simulink library "MatlabHeatLib"  (Simulink 8.6)
settings: Solver=ode45  StartTime=0.0  StopTime=10.0  RelTol=1e-3
undefined symbols (not defined in the file): ts
libraries: MatlabHeatLib x4, simulink x3
settings Model: Creator=Kai  LastModifiedBy=abp412  ModifiedHistory=Version 2.0 09.05.2011 10:37 Aktuelle Version der MatlabHeatLib

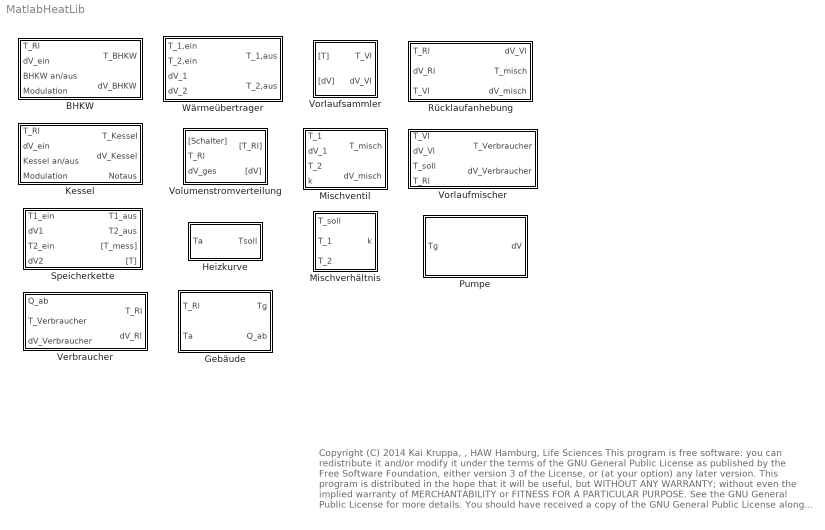
== system MatlabHeatLib ==
  note: Copyright (C) 2014 Kai Kruppa, , HAW Hamburg, Life Sciences
      |
      |     This program is free software: you can redistribute it and/or modify it under the terms of the GNU General Public License
      | as published by the Free Software Foundation, either version 3 of the License, or (at your option) any later version.
      |
      | This program is distributed in the hope that it will be useful, but WITHOUT ANY WARRANTY;
      | without even the implied warranty of MERCHANTABILITY or FITNESS FOR A PARTICULAR PURPOSE.
      | See the GNU General Public License for more details.
      |
      |     You should have received a copy of the GNU General Public License along with this program.  If not, see <http://www.gnu.org/licenses/>.
      |
      | Contact: kai.kruppa@haw-hamburg.de
  BHKW : Subsystem  mask(BHKW){V_BHKW=1.02, P_min=100, P_max=200, k_BHKW=2681, c=4182, rho=1000, BHKWInit=273+70, T_Umgebung=273+30}
      mask prompts: V_BHKW "Volumen [m^3]"; P_min "minimale Leistung [kW]"; P_max "maximale Leistung [kW]"; k_BHKW "Verlustleistungskoeffizient [kW/K]"; c "spez. Wärmekapazität [J/(kg*K)]"; rho "Dichte [kg/m^3]"; BHKWInit "Anfangstemperatur [K]"; T_Umgebung "Umgebungstemperatur [K]"
      mask help:
      | Eingänge:
      | - T_Rl, dV_ein:  Volumenstrom dV_ein mit der Temperatur T_Rl
      | - BHKW an/aus: öffnet und schließt das Ventil des BHKW's
      | - Modulation:     variiert die zugeführte Leistung Q_zu,
      |                         das Signal liegt im Intervall [0,1]
      | Augänge:
      | -T_BHKW, dV_BHKW: Wasser fließt mit einem Volumenstrom
      |                                 dV_BHKW und der Temperatur T_BHKW ab
      | Die Berechnung der Ausgangstemperatur erfolgt über die
      | Wärmeleistungsbilanz:
      | dQ_BHKW = dQ_zu - dQ_Verlust + dQ_BHKW,Rl - dQ_BHKW,Vl
      | Die zugeführte Leistung Q_zu wird auf eine minimale und eine
      | maximale Leistung begrenzt. Ist das BHKW ausgeschaltet, fließt
      | kein Volumenstrom durch die Komponente.
      | Entwickelt auf Grundlage der Bachelorarbeit "Vergleich
      | verschiedener Wärmeversorgungssysteme", 2010 von Herrn Kai
      | Kruppa.
      |
      | Copyright (C) 2014 Kai Kruppa, HAW Hamburg, Life Sciences,
      | GNU General Public License
  Gebäude : Subsystem  mask(Gebäude){kg=0, krg=0, kga=0, TgInit=0}
      mask prompts: kg "Wärmekapazität"; krg "Wärmeübvergnagskoeffizient (Heizung -> Gebäude)"; kga "Wärmeübvergnagskoeffizient (Gebäude -> Umgebung)"; TgInit "Anfangswert der Gebäudetemperatur [K]"
      mask help:
      | Eingänge:
      | - T_Rl: Rücklauftemperatur
      | - Ta:  Außentemperatur
      |
      | Ausgänge:
      | - Tg: Gebäudetemperatur
      | - Q_ab: Wärmeleistungsbedarf
      | Das Gebäude wird als 1 Zonen Modell angenommen. Die
      | Berechnung der Gebäudetemperatur erfolgt über die
      | Wärmeleistungsbilanz
      | kg*dTg = krg(T_Rl-Tg)-kga(Tg-Ta).
      | Der Wärmeleistungsbedarf lautet
      | Q_ab = krg(T_Rl-Tg).
      | Entwickelt auf Grundlage von "Tensor Systems: Multilinear
      | Modeling and Applications", 3rd Int. Conference on Simulation
      | and Modeling Methodologies, Technologies and Applications,
      | 2013, Pangalos, G., Eichler, A., Lichtenberg, G.
      |
      | Copyright (C) 2014 Kai Kruppa, HAW Hamburg, Life Sciences,
      | GNU General Public License
  Heizkurve : Subsystem  mask(Heizkurve){Ta1c=20, Ta2c=-12, Ts1c=60, Ts2c=85}
      mask prompts: Ta1c "Ta1 [°C]"; Ta2c "Ta2 [°C]"; Ts1c "Tsoll1 [°C]"; Ts2c "Tsoll2 [°C]"
      mask help:
      | Eingang:
      | -Ta: Aussentemperatur
      | Ausgang:
      | -Tsoll: Vorlaufsolltemperatur
      | Anhand der Außentemperatur wird über eine gesättigte lineare
      | Heizkurve die Vorlaufsolltemperatur bestimmt. Die Heizkurve wird
      | durch zwei Punkte, die als Parameter angegeben werden,
      | bestimmt.
      |          Tsoll
      |            |
      | Tsoll2 _| _______
      |            |               \
      |            |                  \
      |            |                     \
      | Tsoll1 _|                        \________
      |            |
      |            |_______________________Ta
      |                          |           |
      |                        Ta2        Ta1
      | Entwickelt auf Grundlage der Bachelorarbeit "Vergleich
      | verschiedener Wärmeversorgungssysteme", 2010 von Herrn Kai
      | Kruppa.
      |
      | Copyright (C) 2014 Kai Kruppa, HAW Hamburg, Life Sciences,
      | GNU General Public License
      mask init:
      | Ta1=Ta1c+273.15;
      | Ta2=Ta2c+273.15;
      | Ts1=Ts1c+273.15;
      | Ts2=Ts2c+273.15;
  Kessel : Subsystem  mask(Kessel){V_Kessel=2, P_min=200, P_max=15000, k_Kessel=5000, c=4182, rho=1000, notaustemp=273+95, notauszeit=10, KesselInit=273+70, T_Umgebung=273+30}
      mask prompts: V_Kessel "Volumen [m^3]"; P_min "Minimale Leistung [kW]"; P_max "Maximale Leistung [kW]"; k_Kessel "Verlustleistungsfaktor [W/K]"; c "Spez. Wärmekapazität [J/(kg*K)]"; rho "Dichte [kg/m^3]"; notaustemp "Notaustemperatur [K]"; notauszeit "Notauszeit [s]"; KesselInit "Anfangstemperatur [K]"; T_Umgebung "Umgebungstemperatur [K]"
      mask help:
      | Eingänge:
      | - T_Rl, dV_ein:  Volumenstrom dV_ein mit der Temperatur T_Rl
      | - Kessel an/aus: schaltet die zugeführte Leistung Q_zu an oder ab
      | - Modulation:     variiert die zugeführte Leistung Q_zu,
      |                         das Signal liegt im Intervall [0,1]
      | Augänge:
      | -T_Kessel, dV_Kessel: das erhitzte Wasser fließt mit einem
      |                                  Volumenstrom dV_Kessel und der
      |                                  Temperatur T_Kessel wieder ab
      | -Notaus:                     gibt an, ob der Kessel sich im
      |                                  Notausbetrieb befindet
      | Die Berechnung der Ausgangstemperatur erfolgt über die
      | Wärmeleistungsbilanz:
      | dQ_Kessel = dQ_zu - dQ_Verlust + dQ_Kessel,Rl - dQ_Kessel,Vl
      | Die zugeführte Leistung Q_zu wird auf eine minimale und eine
      | maximale Leistung begrenzt.
      | Sonderfälle:
      | Volumenstrom dV_ein beträgt 0: kein Wasser fließt durch den
      | Kessel -> das im Kessel befindliche Wasser heizt sich auf.
      | Notausbetrieb: T_Kessel > Notaustemperatur -> Q_zu = 0 für
      | die Dauer der Notauszeit.
      | Entwickelt auf Grundlage der Bachelorarbeit "Vergleich
      | verschiedener Wärmeversorgungssysteme", 2010 von Herrn Kai
      | Kruppa.
      |
      | Copyright (C) 2014 Kai Kruppa, HAW Hamburg, Life Sciences,
      | GNU General Public License
  Mischventil : Subsystem  mask(Mischventil){}
      mask help:
      | Es handelt sich um ein 3-Wege-Mischventil.
      | Eingänge:
      | -T_1, dV_1: Temperatur und Volumenstrom des ersten Stromes
      | -T_2:           Temperatur des zweiten Volumenstromes
      | -k:               Mischverhältnis
      | Ausgänge:
      | -T_misch, dV_misch: Temperatur und Volumenstrom des Mischprodukts
      | Dem Volumenstrom dV1 kann, abhängig vom Mischverhältnis k, Wasser
      | aus einem zweiten Volumenstrom dV2 beigemischt werden. Das
      | Mischverhältnis ist auf den Volumenstrom dV1 bezogen.
      | k = dV_2/dV_1
      | Für das Mischprodukt ergibt sich:
      | dV_misch = (1 + k)*dV_1,
      | T_misch = (T_1 + k*T_2)/(1+k).
      | Entwickelt auf Grundlage der Bachelorarbeit "Vergleich verschiedener
      | Wärmeversorgungssysteme", 2010 von Herrn Kai Kruppa.
      |
      | Copyright (C) 2014 Kai Kruppa, HAW Hamburg, Life Sciences,
      | GNU General Public License
  Mischverhältnis : Subsystem  mask(Mischverhältnis){}
      mask help:
      | Eingänge:
      | -T_soll: Vorlaufsolltemperatur
      | -T_1:    Temperatur des Volumenstroms 1
      | -T_2:    Temperatur des Volumenstroms 2
      | Ausgang:
      | -k: Mischverhältnis
      | Es wird berechnet, wieviel Wasser durch den Volumenstrom 2 dem
      | Volumenstrom 1 zugeführt werden muss, um eine gewünschte
      | Temperatur des Mischprodukts zu erhalten. Die gewünschte
      | Temperatur wird durch die Solltemperatur vorgegeben.
      | Das Mischverhältinis k berechnet sich aus
      | k = (T_1-T_soll)/(T_soll-T_2).
      | Entwickelt auf Grundlage der Bachelorarbeit "Vergleich verschiedener
      | Wärmeversorgungssysteme", 2010 von Herrn Kai Kruppa.
      |
      | Copyright (C) 2014 Kai Kruppa, HAW Hamburg, Life Sciences,
      | GNU General Public License
  Pumpe : Subsystem  mask(Pumpe){dVm=0, dVa=0, Tg_soll=0, DeltaTg=0}
      mask prompts: dVm "Mittlerer Volumenstrom [m^3/s]"; dVa "Volumenstromamplitude [m^3/s]"; Tg_soll "Soll-Gebäudetemperatur [K]"; DeltaTg "Sättigungstemperaturdifferenz [K]"
      mask help:
      | Eingang:
      | - Tg: Gebäudetemperatur
      | Ausgang:
      | - dV: Volumenstrom
      | Die Pumpe bestimmt den Volumenstrom in Abhängigkeit von der Differenz zwischen tatsächlicher und Soll-Gebäudetemperatur. Aufgrund der Thermostatventile im Verbraucher entsteht ein linearer Zusammenhang, der sich außerhalb der Sättigungstemperaturdifferenz in Sättigung befindet.
      | dV=
      | dVm - dVa,                     für Tg-Tg_soll > Delta_Tg
      | dVm + dVa/Delta_Tg(Tg-Tg_soll) für -Delta_Tg<Tg-Tg_soll<Delta_Tg
      | dVm + dVa                      für Tg-Tg_soll < Delta_Tg
      | Entwickelt auf Grundlage von "Tensor Systems: Multilinear Modeling and
      | Applications", 3rd Int. Conference on Simulation and Modeling Methodologies, Technologies and Applications, 2013, Pangalos, G., Eichler, A., Lichtenberg, G.
      |
      | Copyright (C) 2014 Kai Kruppa, HAW Hamburg, Life Sciences,
      | GNU General Public License
  Rücklaufanhebung : Subsystem  mask{T_min=273+60}
      mask prompts: T_min "Mindestrücklauftemperatur [K]"
      mask help:
      | Es handelt sich um ein 3-Wege-Mischventil, das in den Rücklauf geschaltet wird.
      | Eingänge:
      | - T_Rl,dV_Rl: Temperatur und Volumenstrom des Rücklaufs
      | - T_Vl: Vorlauftemperatur
      | Ausgänge:
      | - dV_Vl: Vorlaufvolumenstrom
      | - T_misch: Temperatur des Mischprodukts
      | - dV_misch: Volumenstrom des Mischprodukts
      | Dem Rücklauf kann warmes Wasser aus dem Vorlauf beigemischt
      | werden, um die Rücklauftemperatur zu erhöhen. Es kann somit in
      | gewissen Grenzen sichergestellt, dass die Rücklauftemperatur nicht
      | unter eine bestimmte Mindestrücklauftemperatur fällt.
      | Entwickelt auf Grundlage der Bachelorarbeit "Vergleich verschiedener
      | Wärmeversorgungssysteme", 2010 von Herrn Kai Kruppa.
      |
      | Copyright (C) 2014 Kai Kruppa, HAW Hamburg, Life Sciences,
      | GNU General Public License
  Speicherkette : Subsystem  mask(Speicherkette){k=4, n=40, mode=0, Tinit=linspace(50,40,8), Hsensors=[1.285, 0.289], Tenv=273+20, Vtank=0.772, Htank=1.64, Hin=1.469, Hout=0.059, U=9.367, keff=10}
      mask prompts: k "Anzahl der Speichertanks (1 - 10)"; n "Anzahl der Rechenknoten pro Tank (1 - 100)"; mode "Zuflussmodus: '0' feste Position, '1' Schichtladung"; Tinit "Anfangstemperaturen der Sensoren in allen Speichern [K]"; Hsensors "Anschlusshöhen der Temperatursensoren in einem Speicher [m]"; Tenv "Umgebungstemperatur [K]"; Vtank "Volumen jedes Speichers [m^3]"; Htank "Höhe jedes Speichers [m]"; Hin "Anschlusshöhe des Ladezuflusses [m]"; Hout "Anschlusshöhe des Ladeabflusses [m]"; U "Wärmedurchgangskoeffizient [W/(m^2 K)]"; keff "Effektive vertikale Wärmeleitfähigkeit [W/(m K)]"
      mask help:
      | Eingänge:
      | T1_ein: Eingangstemperatur des Vol.stroms 1
      | dV1:     Volumenstrom 1
      | T2_ein: Eingangstemperatur des Vol.stroms 2
      | dV2:     Volumenstrom 2
      | Ausgänge:
      | T1_aus:    Eingangstemperatur des Vol.stroms 1
      | T2_aus:    Eingangstemperatur des Vol.stroms 2
      | [T_mess]: Temperaturen der Messpunkte
      | [T]:          Temperaturen der Speicherschichten
      | Mit dem Speicher kann warmes Wasser gespeichert und zu einem
      | späteren Zeitpunkt zur Verfügung gestellt werden. Die
      | Durchflussrichtung des Speichers ergibt sich aus den Größen
      | von dV1 und dV2. Die Berechnung der
      | Speicherschichttemperaturen erfolgt über ein nichtlineares
      | Modell, dass durch einen integrierten C-Code berechnet wird.
      | Entwickelt auf Grundlage der Masterarbeit "Entwicklung einer
      | nichtlinearen modellprädiktiven Heizungsregelung zur energetisch
      | optimierten Nutzung eines Warmwasserspeichers", 2012 von
      | Herrn Jan Seifert.
      |
      | Copyright (C) 2014 Kai Kruppa, HAW Hamburg, Life Sciences,
      | GNU General Public License
  Verbraucher : Subsystem  mask(Verbraucher){V_Ver=10, c=4182, rho=1000, InitTempVerbr=335}
      mask prompts: V_Ver "Volumen des Verbrauchers [m^3]"; c "spez. Wärmekapazität [J/(kg*K)]"; rho "Dichte [kg/m^3]"; InitTempVerbr "Anfangstemperatur [K]"
      mask help:
      | Eingänge:
      | - Q_ab:                    vom Verbraucher aufgenommene Leistung
      | - T_Verb., dV_Verb.: Volumenstrom dV_Verb. mit der Temperatur
      |                                T_Verb. fließt hinein
      | Ausgänge:
      | - T_Rl, dV_Rl: das Wasser wird durch den Volumenstrom dV_Rl
      |                       mit der Temperatur T_Rl abgeführt
      | Die Ausgangstemperatur des Verbraucher berechnet sich aus der
      | Wärmeleistungsbilanz:
      | dQ_Verbraucher = dQ_Verbraucher,Vl - dQ_Verbraucher,Rl - dQ_ab
      | Entwickelt auf Grundlage der Bachelorarbeit "Vergleich
      | verschiedener Wärmeversorgungssysteme", 2010 von Herrn Kai
      | Kruppa.
      |
      | Copyright (C) 2014 Kai Kruppa, HAW Hamburg, Life Sciences,
      | GNU General Public License
  Volumenstromverteilung : Subsystem  mask(Volumenstromverteilung){}
      mask help:
      | Eingänge:
      | -Schalter: Vektor mit den Schaltersignalen der einzelnen
      |                Wärmeerzeuger
      | -T_Rl:       Temperatur des Rücklaufvolumenstroms
      | -dV_ges:   gesamter Volumenstrom des Rücklaufs
      | Ausgänge:
      | -[T_Rl]: Vektor mit den Rücklauftemperaturen für die Eingänge der
      |              einzelnen Wärmeerzeuger
      | -[dV]:    Vektor mit den dazugehörigen Volumenströmen
      | Anhand der Schaltersignale wird der gesamte Volumenstrom auf die
      | Wärmeerzeuger aufgeteilt. Über die Schaltersignale wird festgelegt, in
      | welchem Verhältnis die Aufteilung erfolgen soll. Dieses Verhältnis kann
      | absolut oder prozentual angegeben werden.
      | Die Temperatur dieser einzelnen Volumenströme ist die des gesamten Rücklaufs.
      | Entwickelt auf Grundlage der Bachelorarbeit "Vergleich verschiedener
      | Wärmeversorgungssysteme", 2010 von Herrn Kai Kruppa.
      |
      | Copyright (C) 2014 Kai Kruppa, HAW Hamburg, Life Sciences,
      | GNU General Public License
  Vorlaufmischer : Subsystem  mask(Vorlaufmischer){}
      mask help:
      | Es handelt sich um ein 3-Wege-Ventil, das zwischen Vor- und Rücklauf
      | geschaltet wird.
      | Eingänge:
      | -T_Vl, dV_Vl: Temperatur und Volumenstrom des Vorlaufs
      | -T_soll:          Vorlaufsolltemperatur
      | -T_Rl:            Temperatur des Rücklaufs
      | Ausgänge:
      | -T_Verb., dV_Verb.: Temperatur und Volumenstrom des Mischprodukts
      | Dem warmen Vorlauf kann kälteres Wasser aus dem Rücklauf
      | beigemischt werden, um eine bestimmte vorgegebene Vorlaufsolltemperatur zu erhalten. Die Solltemperatur
      | muss dazu zwischen der Vor- und der Rücklauftemperatur liegen.
      | Die Ausgangstemperatur kann so in gewissen Maßen begrenzt werden.
      | Entwickelt auf Grundlage der Bachelorarbeit "Vergleich verschiedener
      | Wärmeversorgungssysteme", 2010 von Herrn Kai Kruppa.
      |
      | Copyright (C) 2014 Kai Kruppa, HAW Hamburg, Life Sciences,
      | GNU General Public License
  Vorlaufsammler : Subsystem  mask(Vorlaufsammler){}
      mask help:
      | Knotenpunkt für die ankommenden Volumenströme aus den einzelnen Wärmeerzeugern.
      | Eingänge:
      | -[T]:  Vektor mit den Temperaturen der Volumenströme aus den
      |          Wärmerzeugern
      | -[dV]: Vektor, der die dazugehörigen Volumenströme beinhaltet
      | Ausgänge:
      | -T_Vl:  Temperatur des Vorlaufs
      | -dV_Vl: Vorlaufvolumenstrom
      | Der Volumenstrom des Vorlaufs berechnet sich aus der Addition der ankommenden Volumenströme.
      | dV_Vl = dV1 + dV2 + ... +dVn
      | Die Vorlauftemperatur ergibt sich aus der Wärmeleistungsbilanz am Knotenpunkt.
      | T_Vl = (T1*dV1+T2+dV2+...Tn*dVn)/dV_Vl
      | Entwickelt auf Grundlage der Bachelorarbeit "Vergleich verschiedener
      | Wärmeversorgungssysteme", 2010 von Herrn Kai Kruppa.
      |
      | Copyright (C) 2014 Kai Kruppa, HAW Hamburg, Life Sciences,
      | GNU General Public License
  Wärmeübertrager : Subsystem  mask(Wärmeübertrager){R_f=0.0023, R_inf=0, beta=-1.5e-5, ts=300, rho=1000, c=4182, F=0.14, n=99}
      mask prompts: R_f "Wärmeleitwiderstand [m^2K/W]"; R_inf "Wärmeleitwiderstand für t->inf [m^2K/W]"; beta "Schichtwachstumskoeffizient [1/s]"; ts "Abtastzeit [s]"; rho "Dichte [kg/m^3]"; c "Spez. Wärmekapazität [J/kg K]"; F "Fläche einer Übertragungsplatte"; n "Anzahl der Übertragungsplatten"
      mask help:
      | Eingänge:
      | T_1,ein: Temperatur des einfließenden Vol.stroms (Primärseite)
      | T_2,ein: Temperatur des einfließenden Vol.stroms (Sekundärseite)
      | dV_1:     Volumenstrom auf der Primärseite
      | dV_2:     Volumenstrom auf der Sekundärseite
      | Ausgänge:
      | T_1,aus: Temperatur des ausfließenden Vol.stroms (Primärseite)
      | T_2,aus: Temperatur des ausfließenden Vol.stroms(Sekundärseite)
      | Mit dem Wärmeübertrager kann themische Energie von einem
      | Volumenstrom (Primärseite) auf einen zweiten Volumenstrom
      | übertragen werden. Es handelt sich um einen Gegenstrom-
      | Wärmeübertrager. Die Modellierung erfolgt über Wärmeleistungs-
      | bilanzen, wobei ein statsches Verhalten der Ausgangs-
      | temperaturen vorausgesetzt wird. Somit lassen sich die Ausgangs-
      | temperaturen analytisch berechnen. Außerdem wird der Einfluss
      | der internen Verschmutzung des Wärmeübertragers auf den
      | Wärmeübergangskoeffizienten berücksichtigt.
      | Entwickelt auf Grundlage der Studienarbeit "Modellierung des
      | Wärmetauschers des Bezirksregierungsgebäudes in Düsseldorf",
      | 2011 von Herrn Max Schmidt und der Bachelorarbeit
      | "Modellbildung einer Fernwärmeheizungsanlage und Identifikation
      | der thermischen und hydraulischen Parameter", 2011 von Herrn
      | Timo Spengler.
      |
      | Copyright (C) 2014 Kai Kruppa, HAW Hamburg, Life Sciences,
      | GNU General Public License

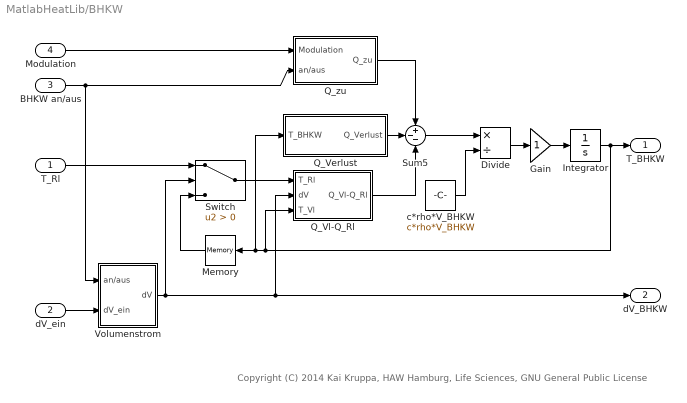
== system MatlabHeatLib/BHKW ==
  note: Copyright (C) 2014 Kai Kruppa, HAW Hamburg, Life Sciences, GNU General Public License
  T_Rl : Inport
  dV_ein : Inport  Port=2
  BHKW an/aus : Inport  Port=3
  Modulation : Inport  Port=4
  Divide : Product  Inputs=*/
  Gain : Gain
  Integrator : Integrator  InitialCondition=BHKWInit  LowerSaturationLimit=273
  Memory : Memory
  Q_Verlust : Subsystem
  Q_Vl-Q_Rl : Subsystem
  Q_zu : Subsystem
  Sum5 : Sum  Inputs=+--
  Switch : Switch  Criteria=u2 > Threshold
  Volumenstrom : Subsystem
  c*rho*V_BHKW : Constant  Value=c*rho*V_BHKW
  T_BHKW : Outport
  dV_BHKW : Outport  Port=2
  wires:
  Volumenstrom/1(dV) -> Q_Vl-Q_Rl/2(dV), dV_BHKW/1, Switch/2
  Integrator/1 -> T_BHKW/1, Q_Vl-Q_Rl/3(T_Vl), Memory/1, Q_Verlust/1(T_BHKW)
  Gain/1 -> Integrator/1
  BHKW an/aus/1 -> Q_zu/2(an/aus), Volumenstrom/1(an/aus)
  Sum5/1 -> Divide/1
  Modulation/1 -> Q_zu/1(Modulation)
  dV_ein/1 -> Volumenstrom/2(dV_ein)
  Q_Verlust/1(Q_Verlust) -> Sum5/2
  Q_Vl-Q_Rl/1(Q_Vl-Q_Rl) -> Sum5/3
  Q_zu/1(Q_zu) -> Sum5/1
  Divide/1 -> Gain/1
  c*rho*V_BHKW/1 -> Divide/2
  T_Rl/1 -> Switch/1
  Switch/1 -> Q_Vl-Q_Rl/1(T_Rl)
  Memory/1 -> Switch/3

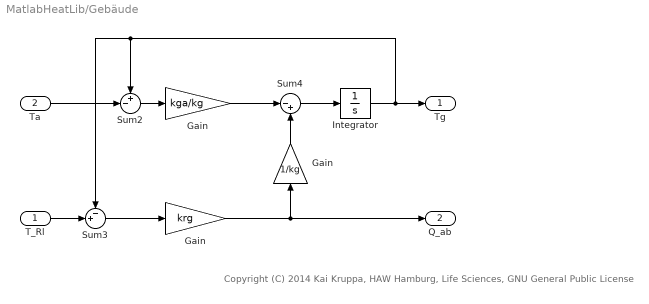
== system MatlabHeatLib/Gebäude ==
  note: Copyright (C) 2014 Kai Kruppa, HAW Hamburg, Life Sciences, GNU General Public License
  T_Rl : Inport
  Ta : Inport  Port=2
  Gain : Gain  Gain=kga/kg
  "Gain " : Gain  Gain=1/kg
  "Gain  " : Gain  Gain=krg
  Integrator : Integrator  InitialCondition=TgInit
  Sum2 : Sum  Inputs=+-|
  Sum3 : Sum  Inputs=-+|
  Sum4 : Sum  Inputs=|-+
  Tg : Outport
  Q_ab : Outport  Port=2
  wires:
  Sum4/1 -> Integrator/1
  "Gain "/1 -> Sum4/2
  "Gain  "/1 -> Q_ab/1, "Gain "/1
  T_Rl/1 -> Sum3/2
  Ta/1 -> Sum2/2
  Sum3/1 -> "Gain  "/1
  Gain/1 -> Sum4/1
  Sum2/1 -> Gain/1
  Integrator/1 -> Sum3/1, Sum2/1, Tg/1

== system MatlabHeatLib/Heizkurve ==
  note: Copyright (C) 2014 Kai Kruppa, HAW Hamburg, Life Sciences, GNU General Public License
  Ta : Inport
  Saturation : Saturate  UpperLimit=Ts2  LowerLimit=Ts1
  Sum : Sum  Inputs=|++
  a : Gain  Gain=(Ts1-Ts2)/(Ta1-Ta2)
  b : Constant  Value=Ts1-(Ts1-Ts2)/(Ta1-Ta2)*Ta1
  Tsoll : Outport
  wires:
  Saturation/1 -> Tsoll/1
  a/1 -> Sum/1
  Sum/1 -> Saturation/1
  b/1 -> Sum/2
  Ta/1 -> a/1

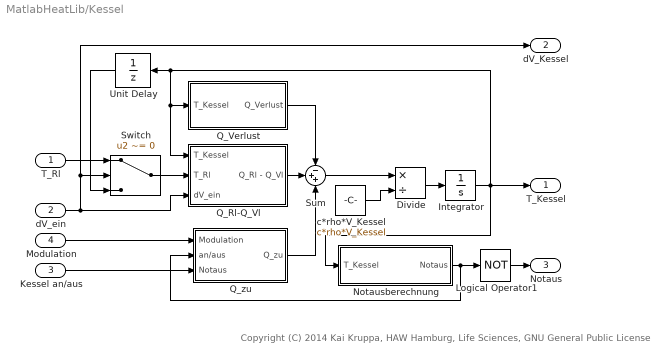
== system MatlabHeatLib/Kessel ==
  note: Copyright (C) 2014 Kai Kruppa, HAW Hamburg, Life Sciences, GNU General Public License
  T_Rl : Inport
  dV_ein : Inport  Port=2
  Kessel an/aus : Inport  Port=3
  Modulation : Inport  Port=4
  Divide : Product  Inputs=*/
  Integrator : Integrator  InitialCondition=KesselInit
  Logical Operator1 : Logic  Operator=NOT  AllPortsSameDT=off  OutDataTypeStr=boolean
  Notausberechnung : Subsystem
  Q_Rl-Q_Vl : Subsystem
  Q_Verlust : Subsystem
  Q_zu : Subsystem
  Sum : Sum  Inputs=-++
  Switch : Switch  Criteria=u2 ~= 0
  Unit Delay : UnitDelay  SampleTime=-1
  c*rho*V_Kessel : Constant  Value=c*rho*V_Kessel
  T_Kessel : Outport
  dV_Kessel : Outport  Port=2
  Notaus : Outport  Port=3
  wires:
  dV_ein/1 -> dV_Kessel/1, Switch/2, Q_Rl-Q_Vl/3(dV_ein)
  Q_zu/1(Q_zu) -> Sum/3
  Q_Verlust/1(Q_Verlust) -> Sum/1
  Q_Rl-Q_Vl/1(Q_Rl - Q_Vl) -> Sum/2
  Sum/1 -> Divide/1
  c*rho*V_Kessel/1 -> Divide/2
  Divide/1 -> Integrator/1
  T_Rl/1 -> Switch/1
  Integrator/1 -> T_Kessel/1, Unit Delay/1, Q_Rl-Q_Vl/1(T_Kessel), Q_Verlust/1(T_Kessel), Notausberechnung/1(T_Kessel)
  Switch/1 -> Q_Rl-Q_Vl/2(T_Rl)
  Unit Delay/1 -> Switch/3
  Notausberechnung/1(Notaus) -> Logical Operator1/1, Q_zu/3(Notaus)
  Logical Operator1/1 -> Notaus/1
  Kessel an/aus/1 -> Q_zu/2(an/aus)
  Modulation/1 -> Q_zu/1(Modulation)

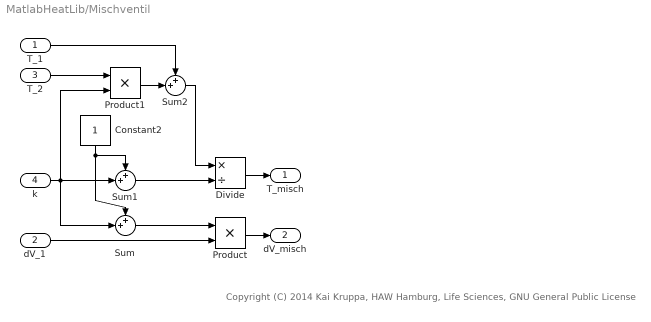
== system MatlabHeatLib/Mischventil ==
  note: Copyright (C) 2014 Kai Kruppa, HAW Hamburg, Life Sciences, GNU General Public License
  T_1 : Inport
  dV_1 : Inport  Port=2
  T_2 : Inport  Port=3
  k : Inport  Port=4
  Constant2 : Constant
  Divide : Product  Inputs=*/
  Product : Product  RndMeth=Zero
  Product1 : Product  RndMeth=Zero
  Sum : Sum  Inputs=++|
  Sum1 : Sum  Inputs=++|
  Sum2 : Sum  Inputs=++|
  T_misch : Outport
  dV_misch : Outport  Port=2
  wires:
  Divide/1 -> T_misch/1
  Sum2/1 -> Divide/1
  Product1/1 -> Sum2/2
  T_1/1 -> Sum2/1
  T_2/1 -> Product1/1
  Sum/1 -> Product/1
  Sum1/1 -> Divide/2
  Constant2/1 -> Sum/1, Sum1/1
  Product/1 -> dV_misch/1
  k/1 -> Product1/2, Sum/2, Sum1/2
  dV_1/1 -> Product/2

== system MatlabHeatLib/Mischverhältnis ==
  note: Copyright (C) 2014 Kai Kruppa, HAW Hamburg, Life Sciences, GNU General Public License
  T_soll : Inport
  T_1 : Inport  Port=2
  T_2 : Inport  Port=3
  Absenkung : Subsystem
  Anhebung : Subsystem
  Relational Operator4 : RelationalOperator  Operator=<  OutDataTypeStr=boolean
  Saturation : Saturate  UpperLimit=1  LowerLimit=0
  Switch4 : Switch  Criteria=u2 > Threshold
  "k " : Subsystem
  k : Outport
  wires:
  Relational Operator4/1 -> Switch4/2
  Absenkung/1(k_ab) -> Switch4/3
  Anhebung/1(k_an) -> Switch4/1
  T_soll/1 -> Relational Operator4/2, "k "/1(T_soll), Absenkung/1(T_soll), Anhebung/1(T_soll)
  T_1/1 -> Relational Operator4/1, "k "/2(T_1), Absenkung/2(T_1), Anhebung/2(T_1)
  T_2/1 -> "k "/3(T_2), Absenkung/3(T_2), Anhebung/3(T_2)
  "k "/1(k) -> Anhebung/4(k), Absenkung/4(k)
  Switch4/1 -> Saturation/1
  Saturation/1 -> k/1

== system MatlabHeatLib/Pumpe ==
  note: Copyright (C) 2014 Kai Kruppa, HAW Hamburg, Life Sciences, GNU General Public License
  Tg : Inport
  Constant : Constant  Value=Tg_soll
  Constant1 : Constant  Value=dVm
  Gain : Gain  Gain=dVa/DeltaTg
  Saturation1 : Saturate  UpperLimit=DeltaTg  LowerLimit=-DeltaTg
  Sum : Sum  Inputs=+-|
  Sum1 : Sum  Inputs=++|
  dV : Outport
  wires:
  Constant1/1 -> Sum1/1
  Sum1/1 -> dV/1
  Gain/1 -> Sum1/2
  Saturation1/1 -> Gain/1
  Sum/1 -> Saturation1/1
  Constant/1 -> Sum/1
  Tg/1 -> Sum/2

== system MatlabHeatLib/Rücklaufanhebung ==
  note: Copyright (C) 2014 Kai Kruppa, HAW Hamburg, Life Sciences, GNU General Public License
  T_Rl : Inport
  dV_Rl : Inport  Port=2
  T_Vl : Inport  Port=3
  Mischventil : MatlabHeatLib/Mischventil
  Mischverhältnis : MatlabHeatLib/Mischverhältnis
  Saturation : Saturate  UpperLimit=inf  LowerLimit=T_min
  dV_Vl : Outport
  T_misch : Outport  Port=2
  dV_misch : Outport  Port=3
  wires:
  Mischventil/2 -> dV_misch/1
  dV_Rl/1 -> dV_Vl/1, Mischventil/2
  Mischventil/1 -> T_misch/1
  Mischverhältnis/1 -> Mischventil/4
  T_Rl/1 -> Mischventil/1, Mischverhältnis/2, Saturation/1
  Saturation/1 -> Mischverhältnis/1
  T_Vl/1 -> Mischventil/3, Mischverhältnis/3

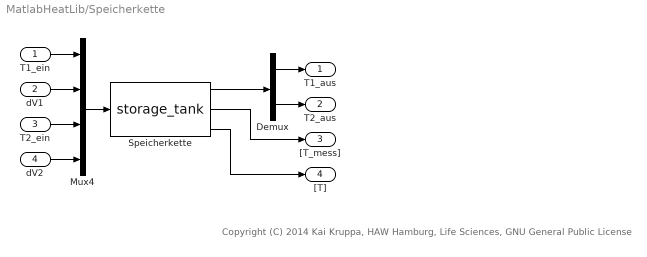
== system MatlabHeatLib/Speicherkette ==
  note: Copyright (C) 2014 Kai Kruppa, HAW Hamburg, Life Sciences, GNU General Public License
  T1_ein : Inport
  dV1 : Inport  Port=2
  T2_ein : Inport  Port=3
  dV2 : Inport  Port=4
  Demux : Demux  Outputs=2
  Mux4 : Mux
  Speicherkette : S-Function  FunctionName=storage_tank  Parameters=mode, n, k, Vtank, Htank, Hin, Hout, U, keff, Tinit, Hsensors, Tenv  SFunctionDeploymentMode=off  EnableBusSupport=off
  T1_aus : Outport
  T2_aus : Outport  Port=2
  "[T_mess]" : Outport  Port=3
  "[T]" : Outport  Port=4
  wires:
  Speicherkette/3 -> "[T]"/1
  Demux/1 -> T1_aus/1
  Demux/2 -> T2_aus/1
  Speicherkette/1 -> Demux/1
  Speicherkette/2 -> "[T_mess]"/1
  Mux4/1 -> Speicherkette/1
  dV2/1 -> Mux4/4
  T2_ein/1 -> Mux4/3
  dV1/1 -> Mux4/2
  T1_ein/1 -> Mux4/1

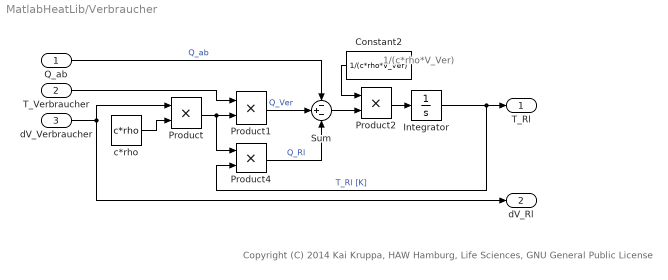
== system MatlabHeatLib/Verbraucher ==
  note: Copyright (C) 2014 Kai Kruppa, HAW Hamburg, Life Sciences, GNU General Public License
  note: 1/(c*rho*V_Ver)
  Q_ab : Inport
  T_Verbraucher : Inport  Port=2
  dV_Verbraucher : Inport  Port=3
  Constant2 : Constant  Value=1/(c*rho*V_Ver)
  Integrator : Integrator  InitialCondition=InitTempVerbr  UpperSaturationLimit=373  LowerSaturationLimit=273
  Product{,1..2,4} (4 alike) : Product  SaturateOnIntegerOverflow=on  RndMeth=Zero  InputSameDT=on  OutDataTypeStr=Inherit: Same as first input
  Sum : Sum  Inputs=-+-  SaturateOnIntegerOverflow=on  InputSameDT=on  OutDataTypeStr=Inherit: Same as first input
  c*rho : Constant  Value=c*rho
  T_Rl : Outport
  dV_Rl : Outport  Port=2
  wires:
  Sum/1 -> Product2/2
  Constant2/1 -> Product2/1
  c*rho/1 -> Product/2
  Q_ab/1 -> Sum/1  "Q_ab"
  Product4/1 -> Sum/3  "Q_Rl"
  Integrator/1 -> Product4/2, T_Rl/1  "T_Rl [K]"
  Product2/1 -> Integrator/1
  Product1/1 -> Sum/2  "Q_Ver"
  Product/1 -> Product4/1, Product1/2
  T_Verbraucher/1 -> Product1/1
  dV_Verbraucher/1 -> Product/1, dV_Rl/1

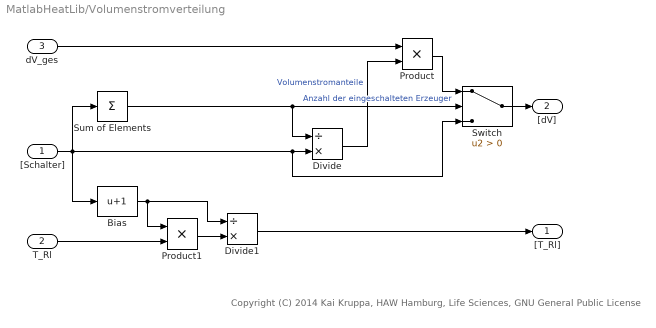
== system MatlabHeatLib/Volumenstromverteilung ==
  note: Copyright (C) 2014 Kai Kruppa, HAW Hamburg, Life Sciences, GNU General Public License
  "[Schalter]" : Inport
  T_Rl : Inport  Port=2
  dV_ges : Inport  Port=3
  Bias : Bias  Bias=1
  Divide : Product  Inputs=/*
  Divide1 : Product  Inputs=/*
  Product : Product  RndMeth=Zero
  Product1 : Product  RndMeth=Zero
  Sum of Elements : Sum  Inputs=+
  Switch : Switch  Criteria=u2 > Threshold
  "[T_Rl]" : Outport
  "[dV]" : Outport  Port=2
  wires:
  "[Schalter]"/1 -> Sum of Elements/1, Bias/1, Divide/2, Switch/3
  dV_ges/1 -> Product/1
  Divide/1 -> Product/2  "Volumenstromanteile"
  Sum of Elements/1 -> Divide/1, Switch/2  "Anzahl der eingeschalteten Erzeuger"
  Bias/1 -> Product1/1, Divide1/1
  T_Rl/1 -> Product1/2
  Product1/1 -> Divide1/2
  Divide1/1 -> "[T_Rl]"/1
  Product/1 -> Switch/1
  Switch/1 -> "[dV]"/1

== system MatlabHeatLib/Vorlaufmischer ==
  note: Copyright (C) 2014 Kai Kruppa, HAW Hamburg, Life Sciences, GNU General Public License
  T_Vl : Inport
  dV_Vl : Inport  Port=2
  T_soll : Inport  Port=3
  T_Rl : Inport  Port=4
  Mischventil : MatlabHeatLib/Mischventil
  Mischverhältnis : MatlabHeatLib/Mischverhältnis
  T_Verbraucher : Outport
  dV_Verbraucher : Outport  Port=2
  wires:
  Mischverhältnis/1 -> Mischventil/4
  Mischventil/1 -> T_Verbraucher/1
  Mischventil/2 -> dV_Verbraucher/1
  T_Vl/1 -> Mischventil/1, Mischverhältnis/2
  dV_Vl/1 -> Mischventil/2
  T_Rl/1 -> Mischventil/3, Mischverhältnis/3
  T_soll/1 -> Mischverhältnis/1

== system MatlabHeatLib/Vorlaufsammler ==
  note: Copyright (C) 2014 Kai Kruppa, HAW Hamburg, Life Sciences, GNU General Public License
  "[T]" : Inport
  "[dV]" : Inport  Port=2
  Constant : Constant  Value=eps
  Divide : Product  Inputs=*/
  Dot Product : DotProduct  InputSameDT=on  OutDataTypeStr=Inherit: Inherit via internal rule
  Memory1 : Memory  X0=273+80
  Sum of Elements : Sum  Inputs=+
  keine Division  durvh '0' : Switch  Criteria=u2 > Threshold  Threshold=eps
  wenn dV=0 -->alter wert : Switch  Criteria=u2 > Threshold
  T_Vl : Outport
  dV_Vl : Outport  Port=2
  wires:
  "[dV]"/1 -> Sum of Elements/1, Dot Product/2
  "[T]"/1 -> Dot Product/1
  Constant/1 -> keine Division  durvh '0'/3
  Sum of Elements/1 -> dV_Vl/1, wenn dV=0 -->alter wert/2, keine Division  durvh '0'/2, keine Division  durvh '0'/1  "dV_Vl"
  Dot Product/1 -> Divide/1
  keine Division  durvh '0'/1 -> Divide/2
  Memory1/1 -> wenn dV=0 -->alter wert/3
  Divide/1 -> wenn dV=0 -->alter wert/1
  wenn dV=0 -->alter wert/1 -> Memory1/1, T_Vl/1

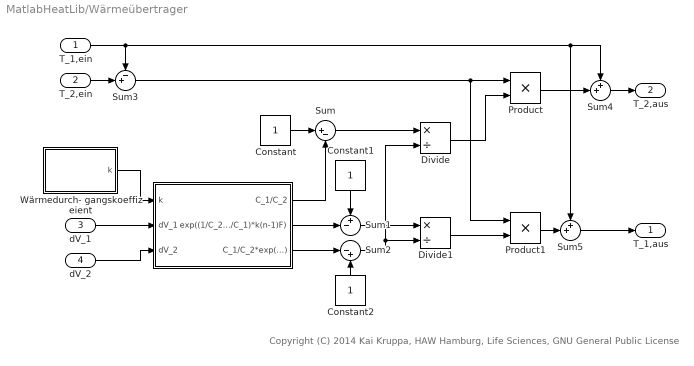
== system MatlabHeatLib/Wärmeübertrager ==
  note: Copyright (C) 2014 Kai Kruppa, HAW Hamburg, Life Sciences, GNU General Public License
  T_1,ein : Inport
  T_2,ein : Inport  Port=2
  dV_1 : Inport  Port=3
  dV_2 : Inport  Port=4
  " " : Subsystem
  Constant : Constant
  Constant1 : Constant
  Constant2 : Constant
  Divide : Product  Inputs=*/
  Divide1 : Product  Inputs=*/
  Product : Product  RndMeth=Zero
  Product1 : Product  RndMeth=Zero
  Sum : Sum  Inputs=|+-
  Sum1 : Sum  Inputs=+-|
  Sum2 : Sum  Inputs=|-+
  Sum3 : Sum  Inputs=-+|
  Sum4 : Sum  Inputs=++|
  Sum5 : Sum  Inputs=++|
  Wärmedurch- gangskoeffizeient : Subsystem
  T_1,aus : Outport
  T_2,aus : Outport  Port=2
  wires:
  Sum5/1 -> T_1,aus/1
  Sum4/1 -> T_2,aus/1
  Product1/1 -> Sum5/2
  Product/1 -> Sum4/2
  Divide1/1 -> Product1/2
  Divide/1 -> Product/2
  Sum3/1 -> Product1/1, Product/1
  T_2,ein/1 -> Sum3/2
  T_1,ein/1 -> Sum5/1, Sum4/1, Sum3/1
  Sum2/1 -> Divide/2, Divide1/2
  Constant2/1 -> Sum2/2
  " "/3(C_1/C_2*exp(...)) -> Sum2/1
  Sum1/1 -> Divide1/1
  Sum/1 -> Divide/1
  Constant1/1 -> Sum1/1
  " "/2(exp((1/C_2-1/C_1)*k(n-1)F)) -> Sum1/2
  Constant/1 -> Sum/1
  " "/1(C_1/C_2) -> Sum/2
  dV_1/1 -> " "/2(dV_1)
  Wärmedurch- gangskoeffizeient/1(k) -> " "/1(k)
  dV_2/1 -> " "/3(dV_2)

== system MatlabHeatLib/BHKW/Q_Verlust ==
  note: Copyright (C) 2014 Kai Kruppa, HAW Hamburg, Life Sciences, GNU General Public License
  T_BHKW : Inport
  Sum : Sum  Inputs=|+-
  T_Umgebung : Constant  Value=T_Umgebung
  "k_BHKW " : Gain  Gain=k_BHKW
  Q_Verlust : Outport
  wires:
  "k_BHKW "/1 -> Q_Verlust/1
  T_BHKW/1 -> Sum/1
  Sum/1 -> "k_BHKW "/1
  T_Umgebung/1 -> Sum/2

== system MatlabHeatLib/BHKW/Q_Vl-Q_Rl ==
  note: Copyright (C) 2014 Kai Kruppa, HAW Hamburg, Life Sciences, GNU General Public License
  T_Rl : Inport
  dV : Inport  Port=2
  T_Vl : Inport  Port=3
  Product2 : Product  RndMeth=Zero
  Sum1 : Sum  Inputs=|-+
  c*rho : Gain  Gain=c*rho
  Q_Vl-Q_Rl : Outport
  wires:
  Product2/1 -> c*rho/1
  Sum1/1 -> Product2/1
  T_Rl/1 -> Sum1/1
  dV/1 -> Product2/2
  T_Vl/1 -> Sum1/2
  c*rho/1 -> Q_Vl-Q_Rl/1

== system MatlabHeatLib/BHKW/Q_zu ==
  note: Copyright (C) 2014 Kai Kruppa, HAW Hamburg, Life Sciences, GNU General Public License
  Modulation : Inport
  an/aus : Inport  Port=2
  P_max : Gain  Gain=P_max*1000
  Product : Product  RndMeth=Zero
  Saturation : Saturate  UpperLimit=P_max*1000  LowerLimit=P_min*1000
  Switch1 : Switch  Criteria=u2 > Threshold
  an : Constant
  aus : Constant  Value=0
  Q_zu : Outport
  wires:
  Switch1/1 -> Product/2
  P_max/1 -> Saturation/1
  Saturation/1 -> Product/1
  aus/1 -> Switch1/3
  an/1 -> Switch1/1
  an/aus/1 -> Switch1/2
  Modulation/1 -> P_max/1
  Product/1 -> Q_zu/1

== system MatlabHeatLib/BHKW/Volumenstrom ==
  note: Copyright (C) 2014 Kai Kruppa, HAW Hamburg, Life Sciences, GNU General Public License
  an/aus : Inport
  dV_ein : Inport  Port=2
  Switch : Switch  Criteria=u2 > Threshold  Threshold=0.5
  ka_BHKW1 : Constant  Value=0
  dV : Outport
  wires:
  ka_BHKW1/1 -> Switch/3
  an/aus/1 -> Switch/2
  dV_ein/1 -> Switch/1
  Switch/1 -> dV/1

== system MatlabHeatLib/Kessel/Notausberechnung ==
  note: Copyright (C) 2014 Kai Kruppa, HAW Hamburg, Life Sciences, GNU General Public License
  T_Kessel : Inport
  Compare To Constant : simulink/Logic and Bit Operations/Compare To Constant  relop=>  const=notaustemp  OutDataTypeStr=uint8
  Compare To Zero : simulink/Logic and Bit Operations/Compare To Zero  relop===  OutDataTypeStr=uint8
  Sum of Elements : Sum  Inputs=+
  Tapped Delay : simulink/Discrete/Tapped Delay  vinit=0.0  samptime=-1  NumDelays=1/ts*notauszeit  DelayOrder=Oldest  includeCurrent=off
  Notaus : Outport
  wires:
  T_Kessel/1 -> Compare To Constant/1
  Tapped Delay/1 -> Sum of Elements/1
  Sum of Elements/1 -> Compare To Zero/1
  Compare To Zero/1 -> Notaus/1
  Compare To Constant/1 -> Tapped Delay/1

== system MatlabHeatLib/Kessel/Q_Rl-Q_Vl ==
  note: Copyright (C) 2014 Kai Kruppa, HAW Hamburg, Life Sciences, GNU General Public License
  T_Kessel : Inport
  T_Rl : Inport  Port=2
  dV_ein : Inport  Port=3
  Product1 : Product  RndMeth=Zero
  Sum : Sum  Inputs=-+|
  c*rho : Gain  Gain=c*rho
  Q_Rl - Q_Vl : Outport
  wires:
  Sum/1 -> c*rho/1
  c*rho/1 -> Product1/1
  T_Kessel/1 -> Sum/1
  T_Rl/1 -> Sum/2
  Product1/1 -> Q_Rl - Q_Vl/1
  dV_ein/1 -> Product1/2

== system MatlabHeatLib/Kessel/Q_Verlust ==
  note: Copyright (C) 2014 Kai Kruppa, HAW Hamburg, Life Sciences, GNU General Public License
  T_Kessel : Inport
  Sum : Sum  Inputs=|+-
  T_Umgebung : Constant  Value=T_Umgebung
  k_Kessel : Gain  Gain=k_Kessel
  Q_Verlust : Outport
  wires:
  T_Umgebung/1 -> Sum/2
  Sum/1 -> k_Kessel/1
  T_Kessel/1 -> Sum/1
  k_Kessel/1 -> Q_Verlust/1

== system MatlabHeatLib/Kessel/Q_zu ==
  note: Copyright (C) 2014 Kai Kruppa, HAW Hamburg, Life Sciences, GNU General Public License
  Modulation : Inport
  an/aus : Inport  Port=2
  Notaus : Inport  Port=3
  Logical Operator : Logic  Inputs=3  AllPortsSameDT=off  OutDataTypeStr=boolean
  P_max : Gain  Gain=P_max * 1000
  Product : Product  RndMeth=Zero
  Saturation : Saturate  UpperLimit=P_max*1000  LowerLimit=P_min*1000
  Q_zu : Outport
  wires:
  Modulation/1 -> P_max/1, Logical Operator/1
  P_max/1 -> Saturation/1
  Saturation/1 -> Product/1
  Logical Operator/1 -> Product/2
  Notaus/1 -> Logical Operator/3
  Product/1 -> Q_zu/1
  an/aus/1 -> Logical Operator/2

== system MatlabHeatLib/Mischverhältnis/Absenkung ==
  note: Copyright (C) 2014 Kai Kruppa, HAW Hamburg, Life Sciences, GNU General Public License
  T_soll : Inport
  T_1 : Inport  Port=2
  T_2 : Inport  Port=3
  k : Inport  Port=4
  Constant : Constant
  Constant1 : Constant  Value=0
  Relational Operator : RelationalOperator  Operator=<=  OutDataTypeStr=boolean
  Relational Operator1 : RelationalOperator  Operator=>  OutDataTypeStr=boolean
  Switch : Switch  Criteria=u2 > Threshold
  Switch1 : Switch  Criteria=u2 > Threshold
  k_ab : Outport
  wires:
  Switch1/1 -> Switch/3
  Constant1/1 -> Switch1/3
  Constant/1 -> Switch1/1
  Relational Operator1/1 -> Switch1/2
  Relational Operator/1 -> Switch/2
  k/1 -> Switch/1
  T_2/1 -> Relational Operator/1, Relational Operator1/2
  T_soll/1 -> Relational Operator/2
  T_1/1 -> Relational Operator1/1
  Switch/1 -> k_ab/1

== system MatlabHeatLib/Mischverhältnis/Anhebung ==
  note: Copyright (C) 2014 Kai Kruppa, HAW Hamburg, Life Sciences, GNU General Public License
  T_soll : Inport
  T_1 : Inport  Port=2
  T_2 : Inport  Port=3
  k : Inport  Port=4
  Constant2 : Constant
  Constant3 : Constant  Value=0
  Relational Operator2 : RelationalOperator  OutDataTypeStr=boolean
  Relational Operator3 : RelationalOperator  Operator=<  OutDataTypeStr=boolean
  Switch2 : Switch  Criteria=u2 > Threshold
  Switch3 : Switch  Criteria=u2 > Threshold
  k_an : Outport
  wires:
  Relational Operator2/1 -> Switch2/2
  Relational Operator3/1 -> Switch3/2
  Constant2/1 -> Switch3/1
  Constant3/1 -> Switch3/3
  Switch3/1 -> Switch2/3
  T_1/1 -> Relational Operator3/1
  k/1 -> Switch2/1
  Switch2/1 -> k_an/1
  T_2/1 -> Relational Operator2/1, Relational Operator3/2
  T_soll/1 -> Relational Operator2/2

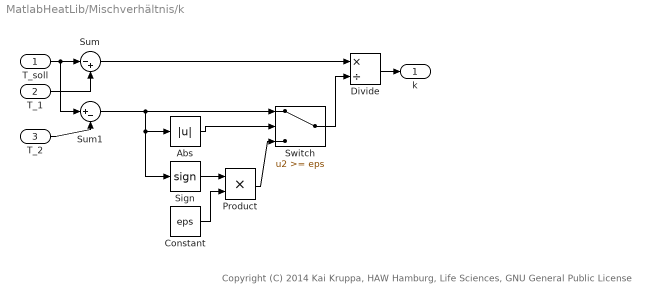
== system MatlabHeatLib/Mischverhältnis/k  ==
  note: Copyright (C) 2014 Kai Kruppa, HAW Hamburg, Life Sciences, GNU General Public License
  T_soll : Inport
  T_1 : Inport  Port=2
  T_2 : Inport  Port=3
  Abs : Abs
  Constant : Constant  Value=eps
  Divide : Product  Inputs=*/
  Product : Product  RndMeth=Zero
  Sign : Signum
  Sum : Sum  Inputs=|-+
  Sum1 : Sum  Inputs=|+-
  Switch : Switch  Threshold=eps
  k : Outport
  wires:
  T_soll/1 -> Sum1/1, Sum/1
  Sum/1 -> Divide/1
  Sum1/1 -> Switch/1, Abs/1, Sign/1
  Abs/1 -> Switch/2
  Sign/1 -> Product/1
  Constant/1 -> Product/2
  Product/1 -> Switch/3
  Switch/1 -> Divide/2
  Divide/1 -> k/1
  T_1/1 -> Sum/2
  T_2/1 -> Sum1/2

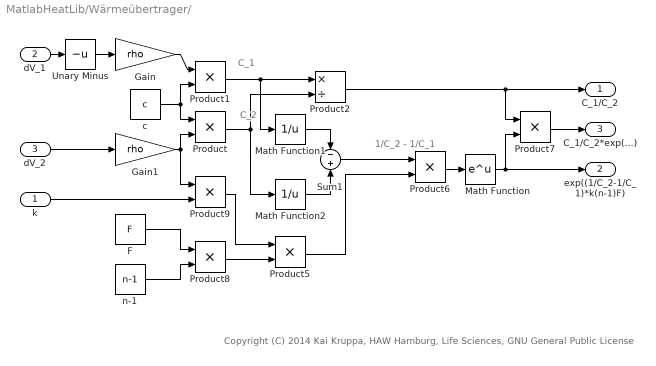
== system MatlabHeatLib/Wärmeübertrager/  ==
  note: Copyright (C) 2014 Kai Kruppa, HAW Hamburg, Life Sciences, GNU General Public License
  note: 1/C_2 - 1/C_1
  note: C_2
  note: C_1
  k : Inport
  dV_1 : Inport  Port=2
  dV_2 : Inport  Port=3
  F : Constant  Value=F
  Gain : Gain  Gain=rho
  Gain1 : Gain  Gain=rho
  Math Function : Math  SaturateOnIntegerOverflow=on
  Math Function1 : Math  Operator=reciprocal  SaturateOnIntegerOverflow=on
  Math Function2 : Math  Operator=reciprocal  SaturateOnIntegerOverflow=on
  Product{,1,5..9} (7 alike) : Product  RndMeth=Zero
  Product2 : Product  Inputs=*/  RndMeth=Zero
  Sum1 : Sum  Inputs=-+
  Unary Minus : UnaryMinus
  c : Constant  Value=c
  n-1 : Constant  Value=n-1
  C_1/C_2 : Outport
  exp((1/C_2-1/C_1)*k(n-1)F) : Outport  Port=2
  C_1/C_2*exp(...) : Outport  Port=3
  wires:
  Math Function1/1 -> Sum1/1
  Gain1/1 -> Product9/1, Product/2
  dV_1/1 -> Unary Minus/1
  Gain/1 -> Product1/1
  Unary Minus/1 -> Gain/1
  k/1 -> Product9/2
  Product9/1 -> Product5/1
  n-1/1 -> Product8/2
  Product8/1 -> Product5/2
  F/1 -> Product8/1
  Product7/1 -> C_1/C_2*exp(...)/1
  Math Function/1 -> exp((1/C_2-1/C_1)*k(n-1)F)/1, Product7/2
  Product2/1 -> C_1/C_2/1, Product7/1
  Product6/1 -> Math Function/1
  Product5/1 -> Product6/2
  Sum1/1 -> Product6/1
  Math Function2/1 -> Sum1/2
  Product/1 -> Math Function2/1, Product2/2
  Product1/1 -> Math Function1/1, Product2/1
  dV_2/1 -> Gain1/1
  c/1 -> Product1/2, Product/1

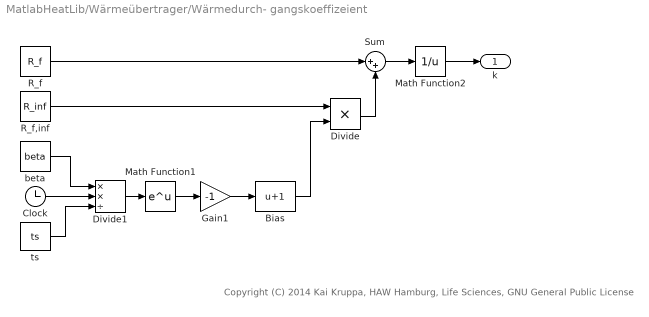
== system MatlabHeatLib/Wärmeübertrager/Wärmedurch- gangskoeffizeient ==
  note: Copyright (C) 2014 Kai Kruppa, HAW Hamburg, Life Sciences, GNU General Public License
  Bias : Bias  Bias=1
  Clock : Clock
  Divide : Product
  Divide1 : Product  Inputs=**/
  Gain1 : Gain  Gain=-1
  Math Function1 : Math  SaturateOnIntegerOverflow=on
  Math Function2 : Math  Operator=reciprocal  SaturateOnIntegerOverflow=on
  R_f : Constant  Value=R_f
  R_f,inf : Constant  Value=R_inf
  Sum : Sum  Inputs=|++
  beta : Constant  Value=beta
  ts : Constant  Value=ts
  k : Outport
  wires:
  beta/1 -> Divide1/1
  R_f,inf/1 -> Divide/1
  R_f/1 -> Sum/1
  Math Function2/1 -> k/1
  ts/1 -> Divide1/3
  Clock/1 -> Divide1/2
  Sum/1 -> Math Function2/1
  Divide/1 -> Sum/2
  Bias/1 -> Divide/2
  Gain1/1 -> Bias/1
  Math Function1/1 -> Gain1/1
  Divide1/1 -> Math Function1/1
